simulink library "qube2servo"  (R2020a)
settings: Solver=VariableStepAuto  StartTime=0.0  StopTime=10.0  RelTol=1e-3
libraries: simulink x6, cstblocks x2
settings Model: Creator=henrik  LastModifiedBy=henrik

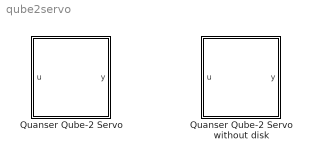
== system qube2servo ==
  Quanser Qube-2 Servo : Subsystem
      mask init:
      | Rm=8.4; %ohm
      | kt=0.042; %Nm/A
      | km=0.042; %V/(rad/s)
      | Jm=4e-6;  %kgm^2
      | Lm=1.16e-3;  %H
      | mh=0.0106; %kg
      | rh=0.0111; %m
      | md=0.053; %kg
      | rd=0.0248; %m
      | 
      | Jh=1/2*mh*rh^2;
      | Jd=1/2*md*rd^2;
      | Jeq=Jm+Jh+Jd; %+Jd;
      | 
      | num=kt/(Jeq*Rm);
      | den=[1 kt*km/(Jeq*Rm) 0];
      | P1=tf(num,den);
      | 
      | Ts=1e-3;
      mask Display: image('$imagefile'); % Use "Edit Image" on toolstrip to change.
  Quanser Qube-2 Servo without disk : Subsystem
      mask init:
      | Rm=8.4; %ohm
      | kt=0.042; %Nm/A
      | km=0.042; %V/(rad/s)
      | Jm=4e-6;  %kgm^2
      | Lm=1.16e-3;  %H
      | mh=0.0106; %kg
      | rh=0.0111; %m
      | md=0; %kg No Disk
      | rd=0.0248; %m
      | 
      | Jh=1/2*mh*rh^2;
      | Jd=1/2*md*rd^2;
      | Jeq=Jm+Jh+Jd; %+Jd;
      | 
      | num=kt/(Jeq*Rm);
      | den=[1 kt*km/(Jeq*Rm) 0];
      | P1=tf(num,den);
      | 
      | Ts=1e-3;
      mask Display: image('$imagefile'); % Use "Edit Image" on toolstrip to change.

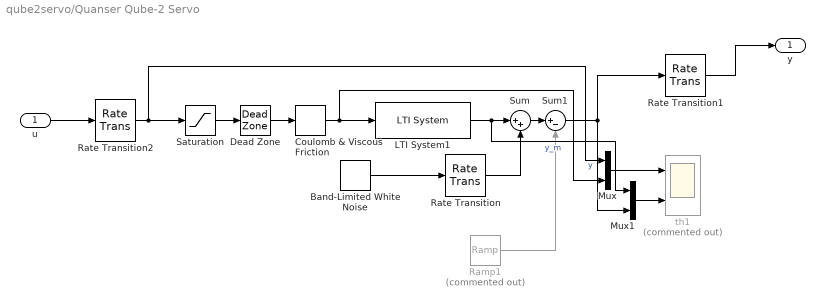
== system qube2servo/Quanser Qube-2 Servo ==
  u : Inport
  Band-Limited White Noise : simulink/Sources/Band-Limited White Noise  Cov=[0.000000001]  Ts=.01  seed=[23341]
  Coulomb & Viscous Friction : simulink/Discontinuities/Coulomb & Viscous Friction  offset=0.2  gain=1
  Dead Zone : DeadZone  LowerValue=-0.2  UpperValue=0.2  SaturateOnIntegerOverflow=on
  LTI System1 : cstblocks/LTI System  sys=P1  IC=[]
  Mux : Mux  Inputs=2
  Mux1 : Mux  Inputs=2
  Ramp1 : simulink/Sources/Ramp  Commented=on  slope=0.1  start=0  InitialOutput=0
  Rate Transition : RateTransition
  Rate Transition1 : RateTransition  OutPortSampleTimeOpt=Inherit  OutPortSampleTime=T
  Rate Transition2 : RateTransition  OutPortSampleTime=Ts
  Saturation : Saturate  UpperLimit=10  LowerLimit=-10
  Sum : Sum  Inputs=|++
  Sum1 : Sum  Inputs=|+-
  th1 : Scope  Commented=on  NumInputPorts=2
  y : Outport
  wires:
  Sum1/1 -> Mux1/2, Rate Transition1/1  "y"
  Ramp1/1 -> Sum1/2
  Coulomb & Viscous Friction/1 -> Mux/2, LTI System1/1
  Sum/1 -> Sum1/1
  LTI System1/1 -> Sum/1, Mux1/1  "y_m"
  Mux1/1 -> th1/2
  Band-Limited White Noise/1 -> Rate Transition/1
  Mux/1 -> th1/1
  Dead Zone/1 -> Coulomb & Viscous Friction/1
  Saturation/1 -> Dead Zone/1
  Rate Transition/1 -> Sum/2
  u/1 -> Rate Transition2/1
  Rate Transition2/1 -> Mux/1, Saturation/1
  Rate Transition1/1 -> y/1

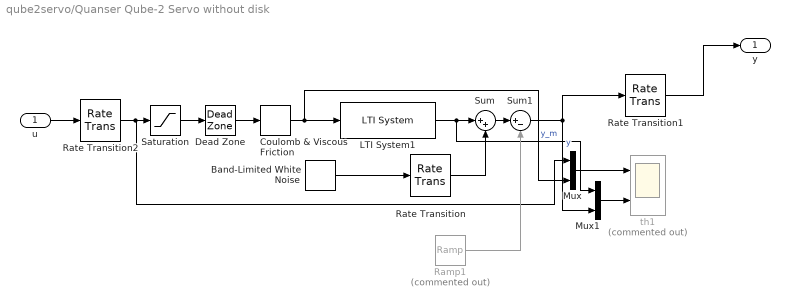
== system qube2servo/Quanser Qube-2 Servo without disk ==
  u : Inport
  Band-Limited White Noise : simulink/Sources/Band-Limited White Noise  Cov=[0.000000001]  Ts=.01  seed=[23341]
  Coulomb & Viscous Friction : simulink/Discontinuities/Coulomb & Viscous Friction  offset=0.2  gain=1
  Dead Zone : DeadZone  LowerValue=-0.2  UpperValue=0.2  SaturateOnIntegerOverflow=on
  LTI System1 : cstblocks/LTI System  sys=P1  IC=[]
  Mux : Mux  Inputs=2
  Mux1 : Mux  Inputs=2
  Ramp1 : simulink/Sources/Ramp  Commented=on  slope=0.1  start=0  InitialOutput=0
  Rate Transition : RateTransition
  Rate Transition1 : RateTransition  OutPortSampleTimeOpt=Inherit  OutPortSampleTime=T
  Rate Transition2 : RateTransition  OutPortSampleTime=Ts
  Saturation : Saturate  UpperLimit=10  LowerLimit=-10
  Sum : Sum  Inputs=|++
  Sum1 : Sum  Inputs=|+-
  th1 : Scope  Commented=on  NumInputPorts=2
  y : Outport
  wires:
  Rate Transition2/1 -> Mux/1, Saturation/1
  Rate Transition/1 -> Sum/2
  Saturation/1 -> Dead Zone/1
  Dead Zone/1 -> Coulomb & Viscous Friction/1
  Mux/1 -> th1/1
  Band-Limited White Noise/1 -> Rate Transition/1
  Mux1/1 -> th1/2
  LTI System1/1 -> Mux1/1, Sum/1  "y_m"
  Sum/1 -> Sum1/1
  Coulomb & Viscous Friction/1 -> LTI System1/1, Mux/2
  Ramp1/1 -> Sum1/2
  Sum1/1 -> Mux1/2, Rate Transition1/1  "y"
  u/1 -> Rate Transition2/1
  Rate Transition1/1 -> y/1
